simulink model "SkywalkerX8_Control_Digital"  (R2018a)
settings: Solver=FixedStepAuto  StartTime=0.0  StopTime=120  FixedStep=0.001  RelTol=1e-3
undefined symbols (not defined in the file): DiscIntNeverNeededParam, sigbuilder_block, SkywalkerX8
libraries: simulink_extras x9, simulink x3
(part 2 of 2)

== system SkywalkerX8_Control_Digital/Autopilot/Gain Scheduled Controller Theta Digital/PDF Controller Theta 2DOF ==
  u : Inport
  P : Inport  Port=2
  D : Inport  Port=3
  N : Inport  Port=4
  Discrete-Time Integrator : DiscreteIntegrator  InitialCondition=SkywalkerX8.InitialConditions.ThetaController.RefController.Derivative  SampleTime=SkywalkerX8.Control.Longitudinal.thetaController.Digital.SampleTime  ICPrevOutput=DiscIntNeverNeededParam  ICPrevScaledInput=DiscIntNeverNeededParam
  POut : Product
  Product : Product
  Product1 : Product
  Sum : Sum  Inputs=|+-
  Sum2 : Sum
  y : Outport  InitialOutput=0
  wires:
  Sum2/1 -> y/1
  N/1 -> Product1/1
  Product1/1 -> Discrete-Time Integrator/1, Sum2/2
  Sum/1 -> Product1/2
  POut/1 -> Sum2/1
  D/1 -> Product/2
  u/1 -> Product/1, POut/2  "u"
  Discrete-Time Integrator/1 -> Sum/2
  Product/1 -> Sum/1
  P/1 -> POut/1

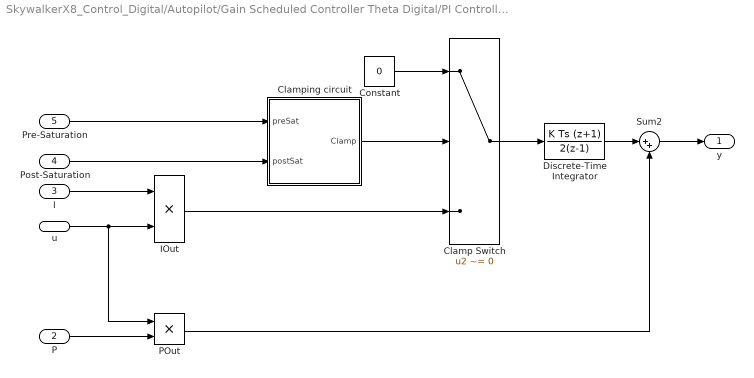
== system SkywalkerX8_Control_Digital/Autopilot/Gain Scheduled Controller Theta Digital/PI Controller Theta ==
  u : Inport
  P : Inport  Port=2
  I : Inport  Port=3
  Post-Saturation : Inport  Port=4
  Pre-Saturation : Inport  Port=5
  Clamp Switch : Switch  Criteria=u2 ~= 0
  Clamping circuit : Subsystem
  Constant : Constant  Value=0
  Discrete-Time Integrator : DiscreteIntegrator  IntegratorMethod=Integration: Trapezoidal  InitialCondition=SkywalkerX8.InitialConditions.ThetaController.Integrator  SampleTime=SkywalkerX8.Control.Longitudinal.thetaController.Digital.SampleTime  ICPrevOutput=DiscIntNeverNeededParam  ICPrevScaledInput=DiscIntNeverNeededParam
  IOut : Product  DisableCoverage=on
  POut : Product
  Sum2 : Sum  Inputs=|++
  y : Outport  InitialOutput=0
  wires:
  IOut/1 -> Clamp Switch/3
  Clamp Switch/1 -> Discrete-Time Integrator/1
  Sum2/1 -> y/1
  Pre-Saturation/1 -> Clamping circuit/1(preSat)
  Post-Saturation/1 -> Clamping circuit/2(postSat)
  Clamping circuit/1(Clamp) -> Clamp Switch/2
  Constant/1 -> Clamp Switch/1
  Discrete-Time Integrator/1 -> Sum2/1
  POut/1 -> Sum2/2
  P/1 -> POut/2
  u/1 -> POut/1, IOut/2
  I/1 -> IOut/1

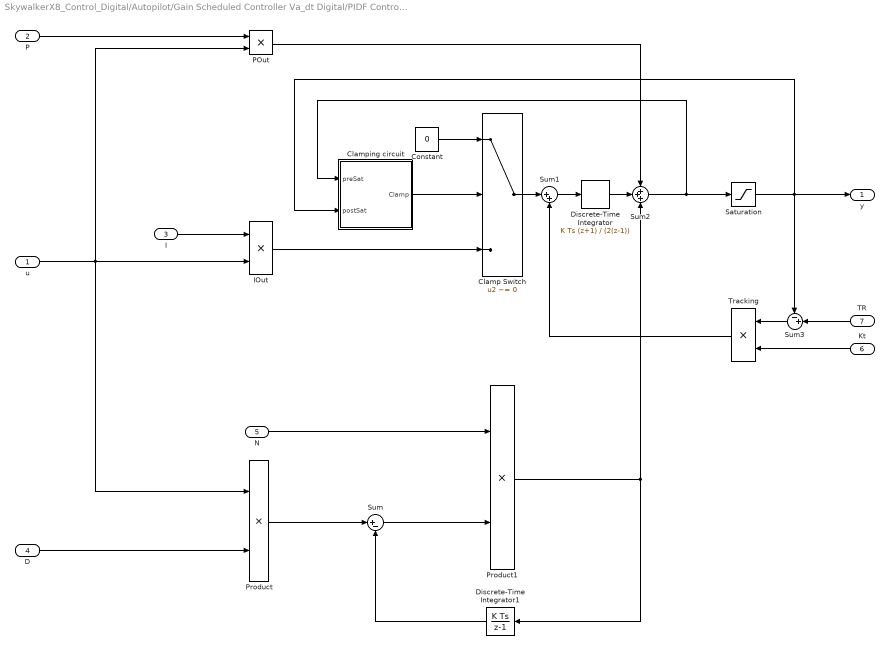
== system SkywalkerX8_Control_Digital/Autopilot/Gain Scheduled Controller Va_dt Digital/PIDF Controller Va_dt ==
  u : Inport
  P : Inport  Port=2
  I : Inport  Port=3
  D : Inport  Port=4
  N : Inport  Port=5
  Kt : Inport  Port=6
  TR : Inport  Port=7
  Clamp Switch : Switch  Criteria=u2 ~= 0
  Clamping circuit : Subsystem
  Constant : Constant  Value=0
  Discrete-Time Integrator : DiscreteIntegrator  IntegratorMethod=Integration: Trapezoidal  InitialCondition=SkywalkerX8.InitialConditions.dt  SampleTime=SkywalkerX8.Control.Longitudinal.VaDtController.Digital.SampleTime  ICPrevOutput=DiscIntNeverNeededParam  ICPrevScaledInput=DiscIntNeverNeededParam
  Discrete-Time Integrator1 : DiscreteIntegrator  SampleTime=SkywalkerX8.Control.Longitudinal.VaDtController.Digital.SampleTime  ICPrevOutput=DiscIntNeverNeededParam  ICPrevScaledInput=DiscIntNeverNeededParam
  IOut : Product  DisableCoverage=on
  POut : Product
  Product : Product
  Product1 : Product
  Saturation : Saturate  UpperLimit=SkywalkerX8.Control.Longitudinal.VaDtController.upperSaturationDt  LowerLimit=SkywalkerX8.Control.Longitudinal.VaDtController.lowerSaturationDt
  Sum : Sum  Inputs=|+-
  Sum1 : Sum  Inputs=|++
  Sum2 : Sum  Inputs=+++
  Sum3 : Sum  Inputs=-+|
  Tracking : Product  DisableCoverage=on
  y : Outport  InitialOutput=0
  wires:
  Saturation/1 -> Clamping circuit/2(postSat), y/1, Sum3/1
  N/1 -> Product1/1
  Product1/1 -> Discrete-Time Integrator1/1, Sum2/3
  Sum2/1 -> Saturation/1, Clamping circuit/1(preSat)
  Sum/1 -> Product1/2
  POut/1 -> Sum2/1
  D/1 -> Product/2
  u/1 -> Product/1, POut/2, IOut/2
  Discrete-Time Integrator1/1 -> Sum/2
  Clamp Switch/1 -> Sum1/1
  Product/1 -> Sum/1
  Discrete-Time Integrator/1 -> Sum2/2
  Constant/1 -> Clamp Switch/1
  I/1 -> IOut/1
  IOut/1 -> Clamp Switch/3
  Clamping circuit/1(Clamp) -> Clamp Switch/2
  P/1 -> POut/1
  TR/1 -> Sum3/2
  Sum3/1 -> Tracking/1
  Kt/1 -> Tracking/2
  Tracking/1 -> Sum1/2
  Sum1/1 -> Discrete-Time Integrator/1

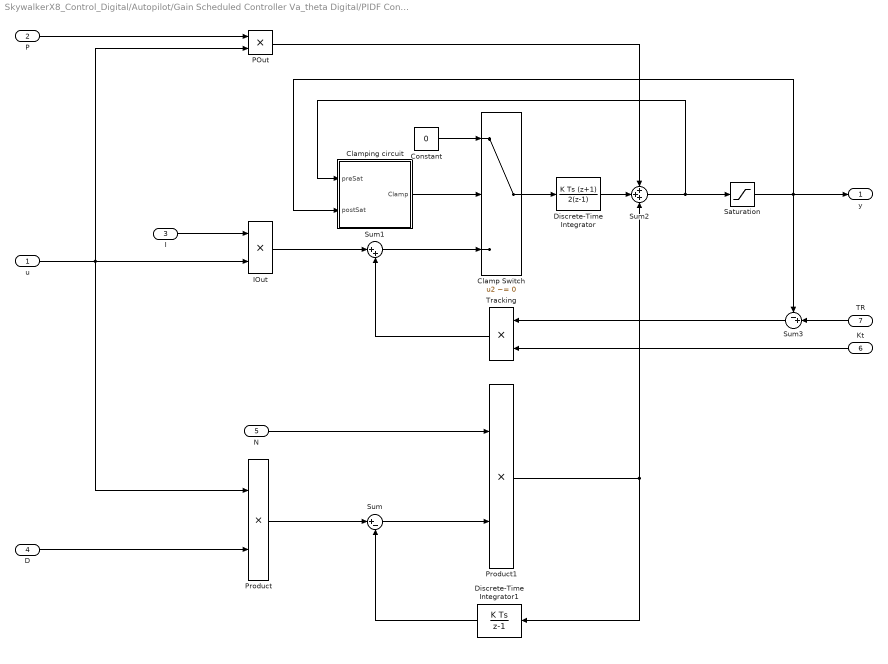
== system SkywalkerX8_Control_Digital/Autopilot/Gain Scheduled Controller Va_theta Digital/PIDF Controller Va_theta ==
  u : Inport
  P : Inport  Port=2
  I : Inport  Port=3
  D : Inport  Port=4
  N : Inport  Port=5
  Kt : Inport  Port=6
  TR : Inport  Port=7
  Clamp Switch : Switch  Criteria=u2 ~= 0
  Clamping circuit : Subsystem
  Constant : Constant  Value=0
  Discrete-Time Integrator : DiscreteIntegrator  IntegratorMethod=Integration: Trapezoidal  InitialCondition=-SkywalkerX8.InitialConditions.PhiThetaPsi(2)  SampleTime=SkywalkerX8.Control.Longitudinal.VaThetaController.Digital.SampleTime  ICPrevOutput=DiscIntNeverNeededParam  ICPrevScaledInput=DiscIntNeverNeededParam
  Discrete-Time Integrator1 : DiscreteIntegrator  SampleTime=SkywalkerX8.Control.Longitudinal.VaThetaController.Digital.SampleTime  ICPrevOutput=DiscIntNeverNeededParam  ICPrevScaledInput=DiscIntNeverNeededParam
  IOut : Product  DisableCoverage=on
  POut : Product
  Product : Product
  Product1 : Product
  Saturation : Saturate  UpperLimit=SkywalkerX8.Control.Longitudinal.VaThetaController.upperSaturationThetaC  LowerLimit=SkywalkerX8.Control.Longitudinal.VaThetaController.lowerSaturationThetaC
  Sum : Sum  Inputs=|+-
  Sum1 : Sum  Inputs=|++
  Sum2 : Sum  Inputs=+++
  Sum3 : Sum  Inputs=-+|
  Tracking : Product  DisableCoverage=on
  y : Outport  InitialOutput=0
  wires:
  Saturation/1 -> Clamping circuit/2(postSat), y/1, Sum3/1
  N/1 -> Product1/1
  Product1/1 -> Discrete-Time Integrator1/1, Sum2/3
  Sum2/1 -> Saturation/1, Clamping circuit/1(preSat)
  Sum/1 -> Product1/2
  POut/1 -> Sum2/1
  D/1 -> Product/2
  u/1 -> Product/1, POut/2, IOut/2
  Discrete-Time Integrator1/1 -> Sum/2
  Clamp Switch/1 -> Discrete-Time Integrator/1
  Product/1 -> Sum/1
  Discrete-Time Integrator/1 -> Sum2/2
  Constant/1 -> Clamp Switch/1
  I/1 -> IOut/1
  Sum1/1 -> Clamp Switch/3
  Clamping circuit/1(Clamp) -> Clamp Switch/2
  P/1 -> POut/1
  IOut/1 -> Sum1/1
  TR/1 -> Sum3/2
  Sum3/1 -> Tracking/1
  Kt/1 -> Tracking/2
  Tracking/1 -> Sum1/2

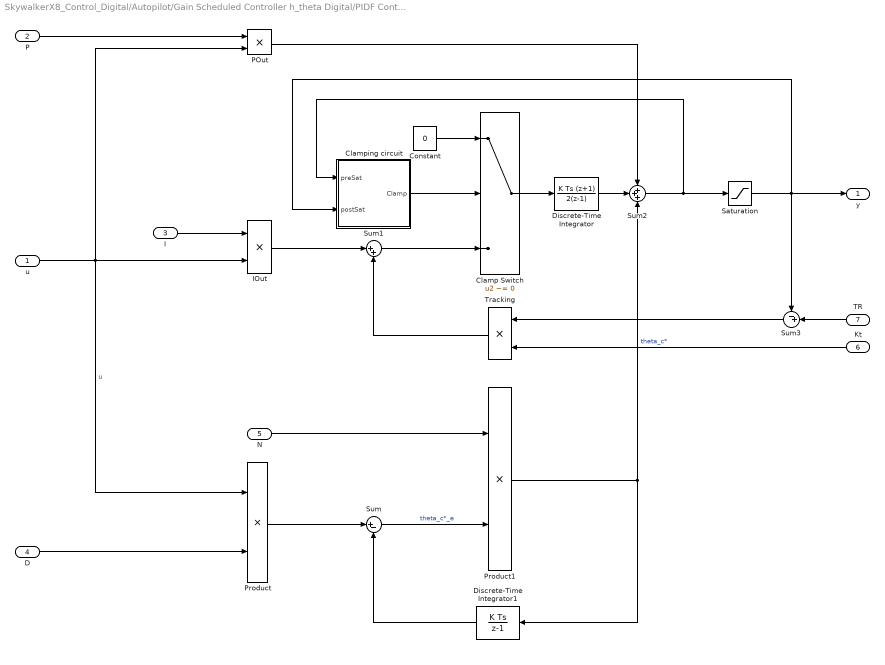
== system SkywalkerX8_Control_Digital/Autopilot/Gain Scheduled Controller h_theta Digital/PIDF Controller h_theta ==
  u : Inport
  P : Inport  Port=2
  I : Inport  Port=3
  D : Inport  Port=4
  N : Inport  Port=5
  Kt : Inport  Port=6
  TR : Inport  Port=7
  Clamp Switch : Switch  Criteria=u2 ~= 0
  Clamping circuit : Subsystem
  Constant : Constant  Value=0
  Discrete-Time Integrator : DiscreteIntegrator  IntegratorMethod=Integration: Trapezoidal  InitialCondition=SkywalkerX8.InitialConditions.PhiThetaPsi(2)  SampleTime=SkywalkerX8.Control.Longitudinal.altController.Digital.SampleTime  ICPrevOutput=DiscIntNeverNeededParam  ICPrevScaledInput=DiscIntNeverNeededParam
  Discrete-Time Integrator1 : DiscreteIntegrator  SampleTime=SkywalkerX8.Control.Longitudinal.altController.Digital.SampleTime  ICPrevOutput=DiscIntNeverNeededParam  ICPrevScaledInput=DiscIntNeverNeededParam
  IOut : Product  DisableCoverage=on
  POut : Product
  Product : Product
  Product1 : Product
  Saturation : Saturate  UpperLimit=SkywalkerX8.Control.Longitudinal.altController.upperSaturationThetaC  LowerLimit=SkywalkerX8.Control.Longitudinal.altController.lowerSaturationThetaC
  Sum : Sum  Inputs=|+-
  Sum1 : Sum  Inputs=|++
  Sum2 : Sum  Inputs=+++
  Sum3 : Sum  Inputs=-+|
  Tracking : Product  DisableCoverage=on
  y : Outport  InitialOutput=0
  wires:
  Saturation/1 -> Clamping circuit/2(postSat), y/1, Sum3/1
  Sum2/1 -> Saturation/1, Clamping circuit/1(preSat)
  POut/1 -> Sum2/1
  Clamp Switch/1 -> Discrete-Time Integrator/1
  Discrete-Time Integrator/1 -> Sum2/2
  Constant/1 -> Clamp Switch/1
  I/1 -> IOut/1
  Sum1/1 -> Clamp Switch/3
  Clamping circuit/1(Clamp) -> Clamp Switch/2
  P/1 -> POut/1
  IOut/1 -> Sum1/1
  TR/1 -> Sum3/2
  Sum3/1 -> Tracking/1
  Kt/1 -> Tracking/2
  Tracking/1 -> Sum1/2
  Discrete-Time Integrator1/1 -> Sum/2
  D/1 -> Product/2
  Product/1 -> Sum/1
  N/1 -> Product1/1
  Product1/1 -> Sum2/3, Discrete-Time Integrator1/1  "theta_c*"
  u/1 -> Product/1, POut/2, IOut/2  "u"
  Sum/1 -> Product1/2  "theta_c*_e"

== system SkywalkerX8_Control_Digital/Autopilot/Gain Scheduled Controller Chi Digital/PIDF Controller Va_theta/Clamping circuit ==
  preSat : Inport  DisableCoverage=on
  postSat : Inport  DisableCoverage=on  Port=2
  Memory : Memory  DisableCoverage=on
  NotEqual : RelationalOperator  DisableCoverage=on  Operator=~=  RndMeth=Nearest  InputSameDT=on
  Clamp : Outport  DisableCoverage=on
  wires:
  postSat/1 -> NotEqual/2
  preSat/1 -> NotEqual/1
  NotEqual/1 -> Memory/1
  Memory/1 -> Clamp/1

== system SkywalkerX8_Control_Digital/Autopilot/Gain Scheduled Controller Phi Digital/PI Controller Phi/Clamping circuit ==
  preSat : Inport  DisableCoverage=on
  postSat : Inport  DisableCoverage=on  Port=2
  Memory : Memory  DisableCoverage=on
  NotEqual : RelationalOperator  DisableCoverage=on  Operator=~=  RndMeth=Nearest  InputSameDT=on
  Clamp : Outport  DisableCoverage=on
  wires:
  postSat/1 -> NotEqual/2
  preSat/1 -> NotEqual/1
  NotEqual/1 -> Memory/1
  Memory/1 -> Clamp/1

== system SkywalkerX8_Control_Digital/Autopilot/Gain Scheduled Controller Theta Digital/PI Controller Theta/Clamping circuit ==
  preSat : Inport  DisableCoverage=on
  postSat : Inport  DisableCoverage=on  Port=2
  Memory : Memory  DisableCoverage=on
  NotEqual : RelationalOperator  DisableCoverage=on  Operator=~=  RndMeth=Nearest  InputSameDT=on
  Clamp : Outport  DisableCoverage=on
  wires:
  postSat/1 -> NotEqual/2
  preSat/1 -> NotEqual/1
  NotEqual/1 -> Memory/1
  Memory/1 -> Clamp/1

== system SkywalkerX8_Control_Digital/Autopilot/Gain Scheduled Controller Va_dt Digital/PIDF Controller Va_dt/Clamping circuit ==
  preSat : Inport  DisableCoverage=on
  postSat : Inport  DisableCoverage=on  Port=2
  Memory : Memory  DisableCoverage=on
  NotEqual : RelationalOperator  DisableCoverage=on  Operator=~=  RndMeth=Nearest  InputSameDT=on
  Clamp : Outport  DisableCoverage=on
  wires:
  postSat/1 -> NotEqual/2
  preSat/1 -> NotEqual/1
  NotEqual/1 -> Memory/1
  Memory/1 -> Clamp/1

== system SkywalkerX8_Control_Digital/Autopilot/Gain Scheduled Controller Va_theta Digital/PIDF Controller Va_theta/Clamping circuit ==
  preSat : Inport  DisableCoverage=on
  postSat : Inport  DisableCoverage=on  Port=2
  Memory : Memory  DisableCoverage=on
  NotEqual : RelationalOperator  DisableCoverage=on  Operator=~=  RndMeth=Nearest  InputSameDT=on
  Clamp : Outport  DisableCoverage=on
  wires:
  postSat/1 -> NotEqual/2
  preSat/1 -> NotEqual/1
  NotEqual/1 -> Memory/1
  Memory/1 -> Clamp/1

== system SkywalkerX8_Control_Digital/Autopilot/Gain Scheduled Controller h_theta Digital/PIDF Controller h_theta/Clamping circuit ==
  preSat : Inport  DisableCoverage=on
  postSat : Inport  DisableCoverage=on  Port=2
  Memory : Memory  DisableCoverage=on
  NotEqual : RelationalOperator  DisableCoverage=on  Operator=~=  RndMeth=Nearest  InputSameDT=on
  Clamp : Outport  DisableCoverage=on
  wires:
  postSat/1 -> NotEqual/2
  preSat/1 -> NotEqual/1
  NotEqual/1 -> Memory/1
  Memory/1 -> Clamp/1

== stateflow chart SkywalkerX8_Control_Digital/Autopilot/Altitude Control State Machine ==
  settings: executeAtInitialization=1
  state Descend_Zone
    during: dt = 0
    during: theta_c = theta_c_Va
  state Altitude_Hold_Zone
    during: dt = dt_Va
    during: theta_c = theta_c_h
  state Landing_Mode
    during: dt = 0
    during: theta_c = theta_c_h
  state Climb_Zone
    during: dt = 1.0
    during: theta_c = theta_c_Va
  state Take_Off_Zone
    during: dt = 1.0
    during: theta_c = theta_c_takeoff
  state Pre_Flight
    during: dt = dt_Va
    during: theta_c = theta_c_h
  Descend_Zone -> Landing_Mode [order 2] : [ h_c == 0 ]
  Altitude_Hold_Zone -> Descend_Zone [order 2] : [h >= (h_c + h_hold*(1+hyst_frac))]
  Descend_Zone -> Altitude_Hold_Zone [order 1] : [h < (h_c + h_hold*(1-hyst_frac))]
  Altitude_Hold_Zone -> Landing_Mode [order 3] : [ h_c == 0 ]
  Pre_Flight -> Altitude_Hold_Zone [order 1] : [PreFlightBypass]
  Climb_Zone -> Altitude_Hold_Zone [order 2] : [h >= (h_c - h_hold*(1+hyst_frac))]
  Altitude_Hold_Zone -> Climb_Zone [order 1] : [h < (h_c - h_hold*(1-hyst_frac))]
  Climb_Zone -> Landing_Mode [order 3] : [ h_c == 0 ]
  Take_Off_Zone -> Landing_Mode [order 2] : [ h_c == 0 ]
  Landing_Mode -> Pre_Flight : [ h == 0 ]
  Take_Off_Zone -> Climb_Zone [order 1] : [h >= h_takeoff*(1+hyst_frac)]
  Climb_Zone -> Take_Off_Zone [order 1] : [h < h_takeoff*(1-hyst_frac)]
  Pre_Flight -> Take_Off_Zone [order 2] : [ h_c > 0 ]
  (default) -> Pre_Flight
  data: dt_Va input; theta_c_Va input; theta_c_h input; h input; h_c input; dt output; theta_c output; h_hold parameter double; theta_c_takeoff parameter double; h_takeoff parameter double; hyst_frac parameter double; PreFlightBypass parameter
